simulink subsystem "mecanic_valva"  (R2022b)
settings: Solver=VariableStepAuto  StartTime=0.0  StopTime=10.0  RelTol=1e-3
values from neighbouring files (symbols this model uses):
  b = 12    [valva_run.m]
  F_dry = 0.5    [valva_run.m]
  k = 6000    [valva_run.m]
  m = 0.03    [valva_run.m]
settings Model: Creator=rus_d  LastModifiedBy=rus_d

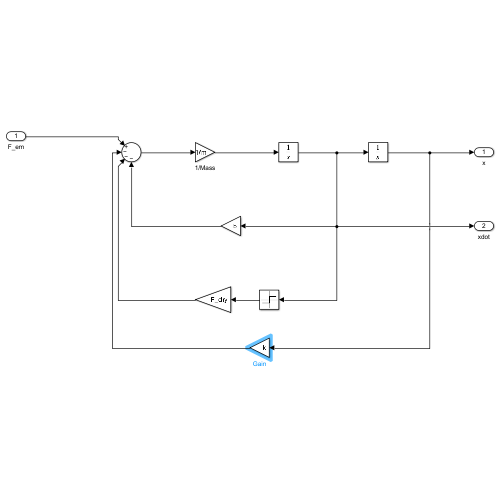
[thumbnail: Simulink's stored preview of the top-level diagram]
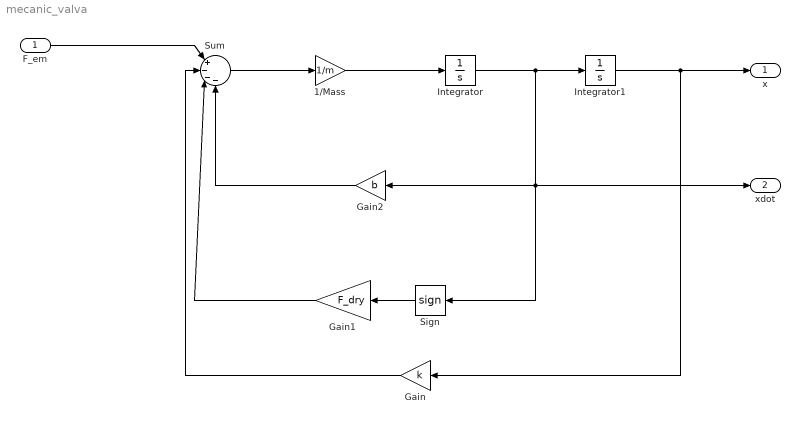
== system mecanic_valva ==
  F_em : Inport
  1/Mass : Gain  Gain=1/m
  Gain : Gain  Gain=k
  Gain1 : Gain  Gain=F_dry
  Gain2 : Gain  Gain=b
  Integrator : Integrator
  Integrator1 : Integrator
  Sign : Signum
  Sum : Sum  Inputs=|+---
  x : Outport
  xdot : Outport  Port=2
  wires:
  F_em/1 -> Sum/1
  Sum/1 -> 1/Mass/1
  1/Mass/1 -> Integrator/1
  Integrator1/1 -> Gain/1, x/1
  Gain/1 -> Sum/2
  Sign/1 -> Gain1/1
  Gain1/1 -> Sum/3
  Gain2/1 -> Sum/4
  Integrator/1 -> Integrator1/1, xdot/1, Gain2/1, Sign/1
